simulink model "freq_planner_example"  (R2020a)
settings: Solver=VariableStepAuto  StartTime=0.0  StopTime=10.0  RelTol=1e-3
libraries: simulink x1, dspsrcs4 x1
settings Model: Creator=jng  LastModifiedBy=jng

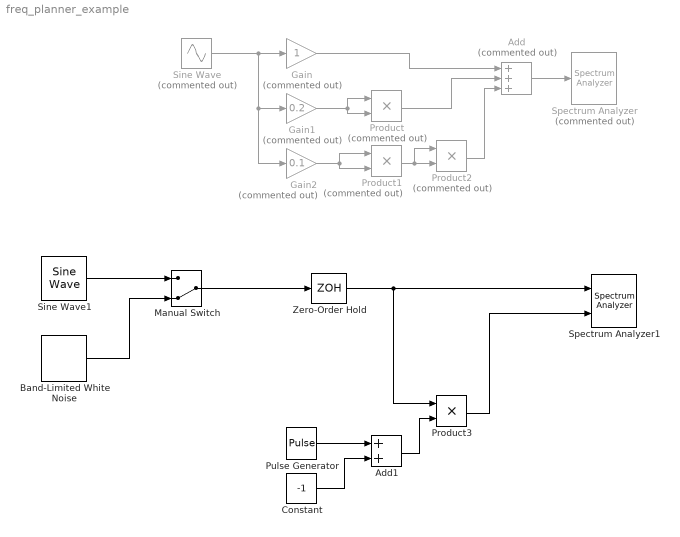
== system freq_planner_example ==
  Add : Sum  Commented=on  Inputs=+++
  Add1 : Sum
  Band-Limited White Noise : simulink/Sources/Band-Limited White Noise  Cov=[0.1]  Ts=1/10e3  seed=[23341]
  Constant : Constant  Value=-1
  Gain : Gain  Commented=on
  Gain1 : Gain  Commented=on  Gain=0.2
  Gain2 : Gain  Commented=on  Gain=0.1
  Manual Switch : ManualSwitch  CurrentSetting=0
  Product : Product  Commented=on
  Product1 : Product  Commented=on
  Product2 : Product  Commented=on
  Product3 : Product
  Pulse Generator : DiscretePulseGenerator  Amplitude=2  Period=10  PulseWidth=5  SampleTime=1/(10*10e3)
  Sine Wave : Sin  Commented=on  Frequency=1575.42  SampleTime=1/4000
  Sine Wave1 : dspsrcs4/Sine Wave  Amplitude=1  Frequency=200  Phase=0  SampleMode=Discrete  OutComplex=Real  CompMethod=Trigonometric fcn  TableSize=Speed  SampleTime=1/10e3  SamplesPerFrame=1  ResetState=Restart at time zero  OutputFrames=off  dataType=double  wordLen=16  udDataType=sfix(16)  fracBitsMode=Best precision  numFracBits=15  OutDataTypeStr=double  LastOutDataTypeStr=double
  Spectrum Analyzer : SpectrumAnalyzer  Commented=on
  Spectrum Analyzer1 : SpectrumAnalyzer  NumInputPorts=2
  Zero-Order Hold : ZeroOrderHold  SampleTime=1/(10*10e3)
  wires:
  Sine Wave/1 -> Gain2/1, Gain1/1, Gain/1
  Gain1/1 -> Product/2, Product/1
  Gain2/1 -> Product1/1, Product1/2
  Product1/1 -> Product2/1, Product2/2
  Add/1 -> Spectrum Analyzer/1
  Gain/1 -> Add/1
  Product/1 -> Add/2
  Product2/1 -> Add/3
  Zero-Order Hold/1 -> Spectrum Analyzer1/1, Product3/1
  Add1/1 -> Product3/2
  Pulse Generator/1 -> Add1/1
  Constant/1 -> Add1/2
  Product3/1 -> Spectrum Analyzer1/2
  Manual Switch/1 -> Zero-Order Hold/1
  Sine Wave1/1 -> Manual Switch/1
  Band-Limited White Noise/1 -> Manual Switch/2
